simulink model "TST_CoME_DemCoord"  (R2016b)
settings: Solver=FixedStepDiscrete  StartTime=0.0  StopTime=simTime  FixedStep=sampleTime  RelTol=1e-3
values from neighbouring files (symbols this model uses):
  testCase = 1    [initTST_CoME_DemCoord_001.m]    (also in initTST_CoME_DemCoord_002.m = 2; initTST_CoME_DemCoord_003.m = 3; initTST_CoME_DemCoord_004.m = 4)
libraries: simulink x29, UnitTest_Lib x24
(part 1 of 2)
settings Model: Creator=zhengjinyan  LastModifiedBy=zhengjinyan
settings DebuggingCC: SignalRangeChecking=error

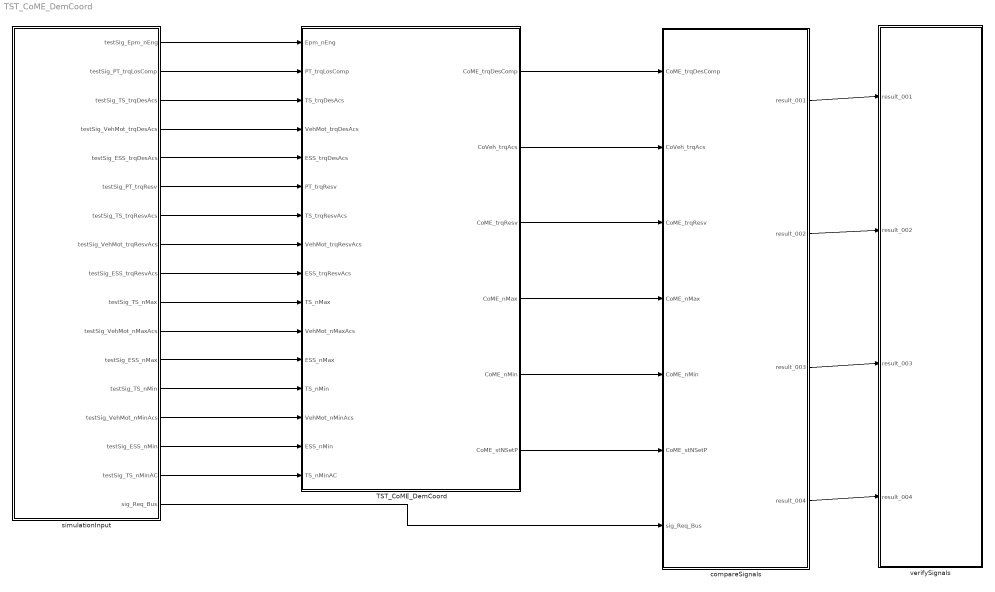
== system TST_CoME_DemCoord ==
  TST_CoME_DemCoord : Subsystem
  compareSignals : Subsystem
  simulationInput : Subsystem
  verifySignals : Subsystem
  wires:
  simulationInput/1(testSig_Epm_nEng) -> TST_CoME_DemCoord/1(Epm_nEng)
  simulationInput/2(testSig_PT_trqLosComp) -> TST_CoME_DemCoord/2(PT_trqLosComp)
  simulationInput/3(testSig_TS_trqDesAcs) -> TST_CoME_DemCoord/3(TS_trqDesAcs)
  simulationInput/4(testSig_VehMot_trqDesAcs) -> TST_CoME_DemCoord/4(VehMot_trqDesAcs)
  simulationInput/5(testSig_ESS_trqDesAcs) -> TST_CoME_DemCoord/5(ESS_trqDesAcs)
  simulationInput/6(testSig_PT_trqResv) -> TST_CoME_DemCoord/6(PT_trqResv)
  simulationInput/7(testSig_TS_trqResvAcs) -> TST_CoME_DemCoord/7(TS_trqResvAcs)
  simulationInput/8(testSig_VehMot_trqResvAcs) -> TST_CoME_DemCoord/8(VehMot_trqResvAcs)
  simulationInput/9(testSig_ESS_trqResvAcs) -> TST_CoME_DemCoord/9(ESS_trqResvAcs)
  simulationInput/10(testSig_TS_nMax) -> TST_CoME_DemCoord/10(TS_nMax)
  simulationInput/11(testSig_VehMot_nMaxAcs) -> TST_CoME_DemCoord/11(VehMot_nMaxAcs)
  simulationInput/12(testSig_ESS_nMax) -> TST_CoME_DemCoord/12(ESS_nMax)
  simulationInput/13(testSig_TS_nMin) -> TST_CoME_DemCoord/13(TS_nMin)
  simulationInput/14(testSig_VehMot_nMinAcs) -> TST_CoME_DemCoord/14(VehMot_nMinAcs)
  simulationInput/15(testSig_ESS_nMin) -> TST_CoME_DemCoord/15(ESS_nMin)
  simulationInput/16(testSig_TS_nMinAC) -> TST_CoME_DemCoord/16(TS_nMinAC)
  TST_CoME_DemCoord/1(CoME_trqDesComp) -> compareSignals/1(CoME_trqDesComp)
  TST_CoME_DemCoord/2(CoVeh_trqAcs) -> compareSignals/2(CoVeh_trqAcs)
  TST_CoME_DemCoord/3(CoME_trqResv) -> compareSignals/3(CoME_trqResv)
  TST_CoME_DemCoord/4(CoME_nMax) -> compareSignals/4(CoME_nMax)
  TST_CoME_DemCoord/5(CoME_nMin) -> compareSignals/5(CoME_nMin)
  TST_CoME_DemCoord/6(CoME_stNSetP) -> compareSignals/6(CoME_stNSetP)
  simulationInput/17(sig_Req_Bus) -> compareSignals/7(sig_Req_Bus)
  compareSignals/1(result_001) -> verifySignals/1(result_001)
  compareSignals/2(result_002) -> verifySignals/2(result_002)
  compareSignals/3(result_003) -> verifySignals/3(result_003)
  compareSignals/4(result_004) -> verifySignals/4(result_004)

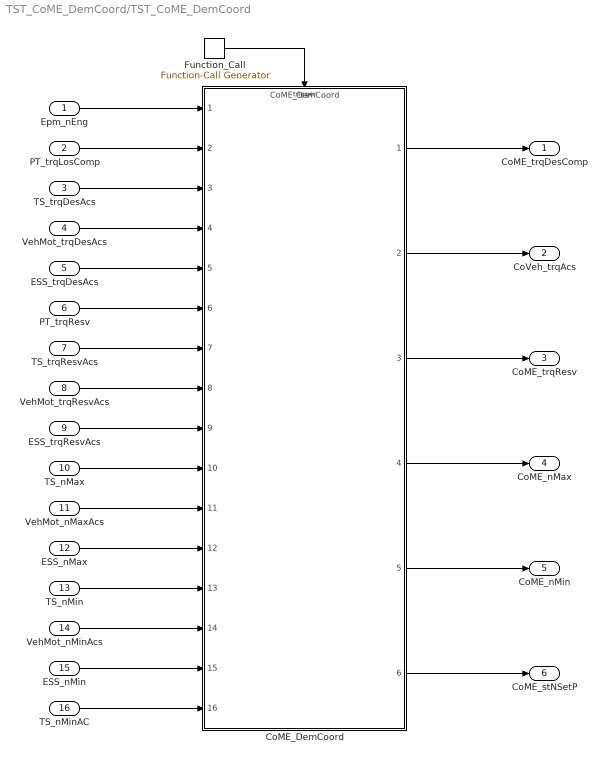
== system TST_CoME_DemCoord/TST_CoME_DemCoord ==
  Epm_nEng : Inport
  PT_trqLosComp : Inport  Port=2
  TS_trqDesAcs : Inport  Port=3
  VehMot_trqDesAcs : Inport  Port=4
  ESS_trqDesAcs : Inport  Port=5
  PT_trqResv : Inport  Port=6
  TS_trqResvAcs : Inport  Port=7
  VehMot_trqResvAcs : Inport  Port=8
  ESS_trqResvAcs : Inport  Port=9
  TS_nMax : Inport  Port=10
  VehMot_nMaxAcs : Inport  Port=11
  ESS_nMax : Inport  Port=12
  TS_nMin : Inport  Port=13
  VehMot_nMinAcs : Inport  Port=14
  ESS_nMin : Inport  Port=15
  TS_nMinAC : Inport  Port=16
  CoME_DemCoord : ModelReference  ModelNameDialog=CoME_DemCoord  SimulationMode=Normal  ModelReferenceVersion=1.11  TriggerPortName=function  TriggerPortTriggerType=function-call  TriggerPortStatesWhenEnabling=held
  Function_Call : simulink/Ports & Subsystems/Function-Call Generator  sample_time=sampleTime  numberOfIterations=1
  CoME_trqDesComp : Outport
  CoVeh_trqAcs : Outport  Port=2
  CoME_trqResv : Outport  Port=3
  CoME_nMax : Outport  Port=4
  CoME_nMin : Outport  Port=5
  CoME_stNSetP : Outport  Port=6
  wires:
  Function_Call/1 -> CoME_DemCoord/Trigger
  Epm_nEng/1 -> CoME_DemCoord/1
  PT_trqLosComp/1 -> CoME_DemCoord/2
  TS_trqDesAcs/1 -> CoME_DemCoord/3
  VehMot_trqDesAcs/1 -> CoME_DemCoord/4
  ESS_trqDesAcs/1 -> CoME_DemCoord/5
  PT_trqResv/1 -> CoME_DemCoord/6
  TS_trqResvAcs/1 -> CoME_DemCoord/7
  VehMot_trqResvAcs/1 -> CoME_DemCoord/8
  ESS_trqResvAcs/1 -> CoME_DemCoord/9
  TS_nMax/1 -> CoME_DemCoord/10
  VehMot_nMaxAcs/1 -> CoME_DemCoord/11
  ESS_nMax/1 -> CoME_DemCoord/12
  TS_nMin/1 -> CoME_DemCoord/13
  VehMot_nMinAcs/1 -> CoME_DemCoord/14
  ESS_nMin/1 -> CoME_DemCoord/15
  TS_nMinAC/1 -> CoME_DemCoord/16
  CoME_DemCoord/1 -> CoME_trqDesComp/1
  CoME_DemCoord/2 -> CoVeh_trqAcs/1
  CoME_DemCoord/3 -> CoME_trqResv/1
  CoME_DemCoord/4 -> CoME_nMax/1
  CoME_DemCoord/5 -> CoME_nMin/1
  CoME_DemCoord/6 -> CoME_stNSetP/1

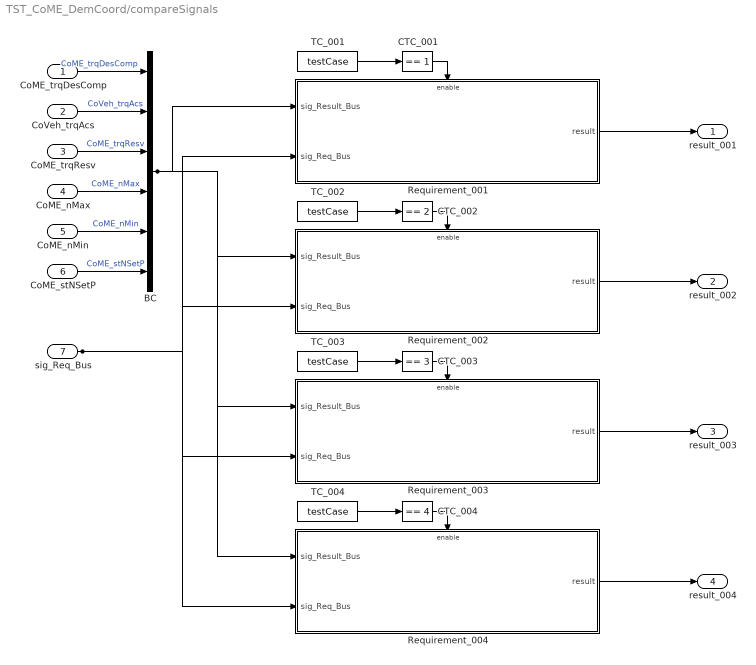
== system TST_CoME_DemCoord/compareSignals ==
  CoME_trqDesComp : Inport
  CoVeh_trqAcs : Inport  Port=2
  CoME_trqResv : Inport  Port=3
  CoME_nMax : Inport  Port=4
  CoME_nMin : Inport  Port=5
  CoME_stNSetP : Inport  Port=6
  sig_Req_Bus : Inport  Port=7
  BC : BusCreator  Inputs=6
  CTC_001 : simulink/Logic and Bit Operations/Compare To Constant  relop===  const=1  OutDataTypeStr=boolean
  CTC_002 : simulink/Logic and Bit Operations/Compare To Constant  relop===  const=2  OutDataTypeStr=boolean
  CTC_003 : simulink/Logic and Bit Operations/Compare To Constant  relop===  const=3  OutDataTypeStr=boolean
  CTC_004 : simulink/Logic and Bit Operations/Compare To Constant  relop===  const=4  OutDataTypeStr=boolean
  Requirement_001 : Subsystem
  Requirement_002 : Subsystem
  Requirement_003 : Subsystem
  Requirement_004 : Subsystem
  TC_001 : Constant  Value=testCase
  TC_002 : Constant  Value=testCase
  TC_003 : Constant  Value=testCase
  TC_004 : Constant  Value=testCase
  result_001 : Outport
  result_002 : Outport  Port=2
  result_003 : Outport  Port=3
  result_004 : Outport  Port=4
  wires:
  CoME_trqDesComp/1 -> BC/1  "CoME_trqDesComp"
  CoVeh_trqAcs/1 -> BC/2  "CoVeh_trqAcs"
  CoME_trqResv/1 -> BC/3  "CoME_trqResv"
  CoME_nMax/1 -> BC/4  "CoME_nMax"
  CoME_nMin/1 -> BC/5  "CoME_nMin"
  CoME_stNSetP/1 -> BC/6  "CoME_stNSetP"
  TC_001/1 -> CTC_001/1
  CTC_001/1 -> Requirement_001/Enable
  sig_Req_Bus/1 -> Requirement_001/2(sig_Req_Bus), Requirement_002/2(sig_Req_Bus), Requirement_003/2(sig_Req_Bus), Requirement_004/2(sig_Req_Bus)
  BC/1 -> Requirement_001/1(sig_Result_Bus), Requirement_002/1(sig_Result_Bus), Requirement_003/1(sig_Result_Bus), Requirement_004/1(sig_Result_Bus)
  Requirement_001/1(result) -> result_001/1
  TC_002/1 -> CTC_002/1
  CTC_002/1 -> Requirement_002/Enable
  Requirement_002/1(result) -> result_002/1
  TC_003/1 -> CTC_003/1
  CTC_003/1 -> Requirement_003/Enable
  Requirement_003/1(result) -> result_003/1
  TC_004/1 -> CTC_004/1
  CTC_004/1 -> Requirement_004/Enable
  Requirement_004/1(result) -> result_004/1

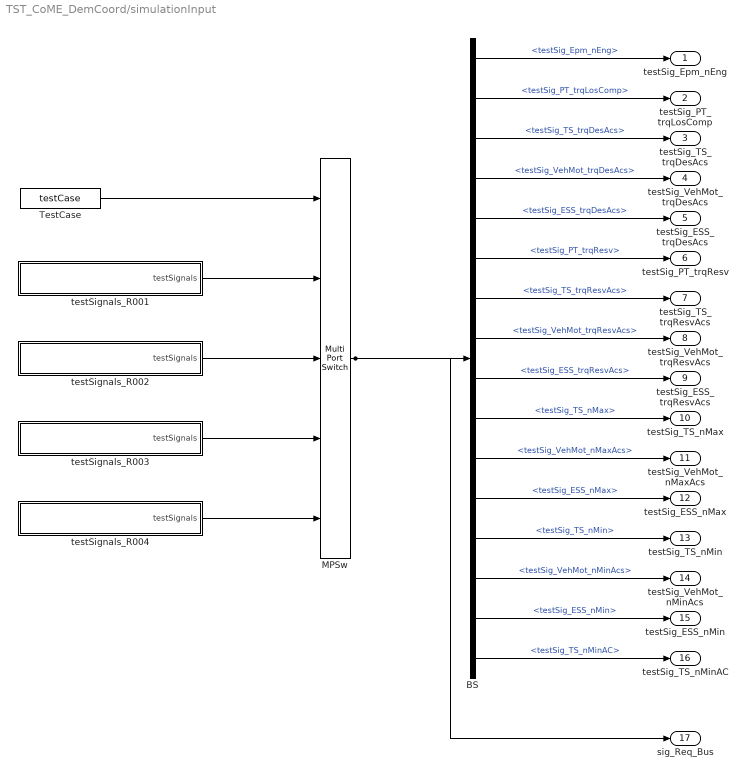
== system TST_CoME_DemCoord/simulationInput ==
  BS : BusSelector  OutputSignals=testSig_Epm_nEng,testSig_PT_trqLosComp,testSig_TS_trqDesAcs,testSig_VehMot_trqDesAcs,testSig_ESS_trqDesAcs,testSig_PT_trqResv,testSig_TS_trqResvAcs,testSig_VehMot_trqResvAcs,testSig_ESS_trqResvAcs,testSig_TS_nMax,testSig_VehMot_nMaxAcs,testSig_ESS_nMax,testSig_TS_nMin,testSig_VehMot_nMinAcs,testSig_ESS_nMin,testSig_TS_nMinAC
  MPSw : MultiPortSwitch  Inputs=4  SaturateOnIntegerOverflow=on  InputSameDT=on
  TestCase : Constant  Value=testCase
  testSignals_R001 : Subsystem
  testSignals_R002 : Subsystem
  testSignals_R003 : Subsystem
  testSignals_R004 : Subsystem
  testSig_Epm_nEng : Outport
  testSig_PT_trqLosComp : Outport  Port=2
  testSig_TS_trqDesAcs : Outport  Port=3
  testSig_VehMot_trqDesAcs : Outport  Port=4
  testSig_ESS_trqDesAcs : Outport  Port=5
  testSig_PT_trqResv : Outport  Port=6
  testSig_TS_trqResvAcs : Outport  Port=7
  testSig_VehMot_trqResvAcs : Outport  Port=8
  testSig_ESS_trqResvAcs : Outport  Port=9
  testSig_TS_nMax : Outport  Port=10
  testSig_VehMot_nMaxAcs : Outport  Port=11
  testSig_ESS_nMax : Outport  Port=12
  testSig_TS_nMin : Outport  Port=13
  testSig_VehMot_nMinAcs : Outport  Port=14
  testSig_ESS_nMin : Outport  Port=15
  testSig_TS_nMinAC : Outport  Port=16
  sig_Req_Bus : Outport  Port=17
  wires:
  BS/1 -> testSig_Epm_nEng/1  "<testSig_Epm_nEng>"
  BS/2 -> testSig_PT_trqLosComp/1  "<testSig_PT_trqLosComp>"
  BS/3 -> testSig_TS_trqDesAcs/1  "<testSig_TS_trqDesAcs>"
  BS/4 -> testSig_VehMot_trqDesAcs/1  "<testSig_VehMot_trqDesAcs>"
  BS/5 -> testSig_ESS_trqDesAcs/1  "<testSig_ESS_trqDesAcs>"
  BS/6 -> testSig_PT_trqResv/1  "<testSig_PT_trqResv>"
  BS/7 -> testSig_TS_trqResvAcs/1  "<testSig_TS_trqResvAcs>"
  BS/8 -> testSig_VehMot_trqResvAcs/1  "<testSig_VehMot_trqResvAcs>"
  BS/9 -> testSig_ESS_trqResvAcs/1  "<testSig_ESS_trqResvAcs>"
  BS/10 -> testSig_TS_nMax/1  "<testSig_TS_nMax>"
  BS/11 -> testSig_VehMot_nMaxAcs/1  "<testSig_VehMot_nMaxAcs>"
  BS/12 -> testSig_ESS_nMax/1  "<testSig_ESS_nMax>"
  BS/13 -> testSig_TS_nMin/1  "<testSig_TS_nMin>"
  BS/14 -> testSig_VehMot_nMinAcs/1  "<testSig_VehMot_nMinAcs>"
  BS/15 -> testSig_ESS_nMin/1  "<testSig_ESS_nMin>"
  BS/16 -> testSig_TS_nMinAC/1  "<testSig_TS_nMinAC>"
  MPSw/1 -> BS/1, sig_Req_Bus/1
  TestCase/1 -> MPSw/1
  testSignals_R001/1(testSignals) -> MPSw/2
  testSignals_R002/1(testSignals) -> MPSw/3
  testSignals_R003/1(testSignals) -> MPSw/4
  testSignals_R004/1(testSignals) -> MPSw/5

== system TST_CoME_DemCoord/verifySignals ==
  result_001 : Inport
  result_002 : Inport  Port=2
  result_003 : Inport  Port=3
  result_004 : Inport  Port=4
  Assertion_001 : Assertion  Enabled=off
  Assertion_002 : Assertion  Enabled=off
  Assertion_003 : Assertion  Enabled=off
  Assertion_004 : Assertion  Enabled=off
  wires:
  result_001/1 -> Assertion_001/1
  result_002/1 -> Assertion_002/1
  result_003/1 -> Assertion_003/1
  result_004/1 -> Assertion_004/1

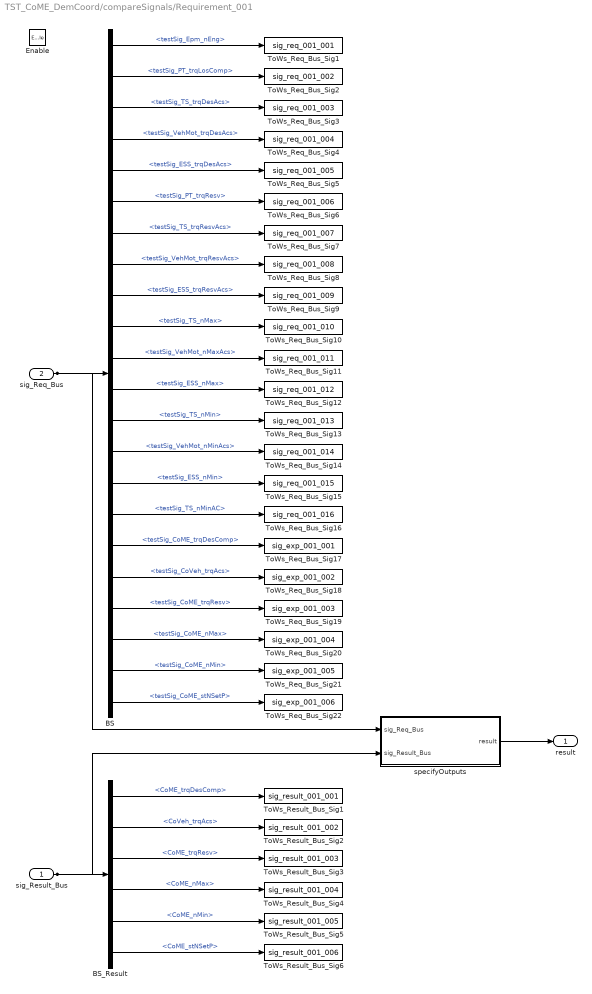
== system TST_CoME_DemCoord/compareSignals/Requirement_001 ==
  sig_Result_Bus : Inport
  sig_Req_Bus : Inport  Port=2
  Enable : EnablePort
  BS : BusSelector  OutputSignals=testSig_Epm_nEng,testSig_PT_trqLosComp,testSig_TS_trqDesAcs,testSig_VehMot_trqDesAcs,testSig_ESS_trqDesAcs,testSig_PT_trqResv,testSig_TS_trqResvAcs,testSig_VehMot_trqResvAcs,testSig_ESS_trqResvAcs,testSig_TS_nMax,testSig_VehMot_nMaxAcs,testSig_ESS_nMax,testSig_TS_nMin,testSig_VehMot_nMinAcs,testSig_ESS_nMin,testSig_TS_nMinAC,testSig_CoME_trqDesComp,testSig_CoVeh_trqAcs,testSig_CoME_trqResv,testSig_CoME_nMax,testSig_CoME_nMin,testSig_CoME_stNSetP
  BS_Result : BusSelector  OutputSignals=CoME_trqDesComp,CoVeh_trqAcs,CoME_trqResv,CoME_nMax,CoME_nMin,CoME_stNSetP
  ToWs_Req_Bus_Sig1 : ToWorkspace  VariableName=sig_req_001_001  SaveFormat=Structure With Time
  ToWs_Req_Bus_Sig10 : ToWorkspace  VariableName=sig_req_001_010  SaveFormat=Structure With Time
  ToWs_Req_Bus_Sig11 : ToWorkspace  VariableName=sig_req_001_011  SaveFormat=Structure With Time
  ToWs_Req_Bus_Sig12 : ToWorkspace  VariableName=sig_req_001_012  SaveFormat=Structure With Time
  ToWs_Req_Bus_Sig13 : ToWorkspace  VariableName=sig_req_001_013  SaveFormat=Structure With Time
  ToWs_Req_Bus_Sig14 : ToWorkspace  VariableName=sig_req_001_014  SaveFormat=Structure With Time
  ToWs_Req_Bus_Sig15 : ToWorkspace  VariableName=sig_req_001_015  SaveFormat=Structure With Time
  ToWs_Req_Bus_Sig16 : ToWorkspace  VariableName=sig_req_001_016  SaveFormat=Structure With Time
  ToWs_Req_Bus_Sig17 : ToWorkspace  VariableName=sig_exp_001_001  SaveFormat=Structure With Time
  ToWs_Req_Bus_Sig18 : ToWorkspace  VariableName=sig_exp_001_002  SaveFormat=Structure With Time
  ToWs_Req_Bus_Sig19 : ToWorkspace  VariableName=sig_exp_001_003  SaveFormat=Structure With Time
  ToWs_Req_Bus_Sig2 : ToWorkspace  VariableName=sig_req_001_002  SaveFormat=Structure With Time
  ToWs_Req_Bus_Sig20 : ToWorkspace  VariableName=sig_exp_001_004  SaveFormat=Structure With Time
  ToWs_Req_Bus_Sig21 : ToWorkspace  VariableName=sig_exp_001_005  SaveFormat=Structure With Time
  ToWs_Req_Bus_Sig22 : ToWorkspace  VariableName=sig_exp_001_006  SaveFormat=Structure With Time
  ToWs_Req_Bus_Sig3 : ToWorkspace  VariableName=sig_req_001_003  SaveFormat=Structure With Time
  ToWs_Req_Bus_Sig4 : ToWorkspace  VariableName=sig_req_001_004  SaveFormat=Structure With Time
  ToWs_Req_Bus_Sig5 : ToWorkspace  VariableName=sig_req_001_005  SaveFormat=Structure With Time
  ToWs_Req_Bus_Sig6 : ToWorkspace  VariableName=sig_req_001_006  SaveFormat=Structure With Time
  ToWs_Req_Bus_Sig7 : ToWorkspace  VariableName=sig_req_001_007  SaveFormat=Structure With Time
  ToWs_Req_Bus_Sig8 : ToWorkspace  VariableName=sig_req_001_008  SaveFormat=Structure With Time
  ToWs_Req_Bus_Sig9 : ToWorkspace  VariableName=sig_req_001_009  SaveFormat=Structure With Time
  ToWs_Result_Bus_Sig1 : ToWorkspace  VariableName=sig_result_001_001  SaveFormat=Structure With Time
  ToWs_Result_Bus_Sig2 : ToWorkspace  VariableName=sig_result_001_002  SaveFormat=Structure With Time
  ToWs_Result_Bus_Sig3 : ToWorkspace  VariableName=sig_result_001_003  SaveFormat=Structure With Time
  ToWs_Result_Bus_Sig4 : ToWorkspace  VariableName=sig_result_001_004  SaveFormat=Structure With Time
  ToWs_Result_Bus_Sig5 : ToWorkspace  VariableName=sig_result_001_005  SaveFormat=Structure With Time
  ToWs_Result_Bus_Sig6 : ToWorkspace  VariableName=sig_result_001_006  SaveFormat=Structure With Time
  specifyOutputs : Subsystem
  result : Outport
  wires:
  sig_Req_Bus/1 -> BS/1, specifyOutputs/1(sig_Req_Bus)
  BS/1 -> ToWs_Req_Bus_Sig1/1  "<testSig_Epm_nEng>"
  BS/2 -> ToWs_Req_Bus_Sig2/1  "<testSig_PT_trqLosComp>"
  BS/3 -> ToWs_Req_Bus_Sig3/1  "<testSig_TS_trqDesAcs>"
  BS/4 -> ToWs_Req_Bus_Sig4/1  "<testSig_VehMot_trqDesAcs>"
  BS/5 -> ToWs_Req_Bus_Sig5/1  "<testSig_ESS_trqDesAcs>"
  BS/6 -> ToWs_Req_Bus_Sig6/1  "<testSig_PT_trqResv>"
  BS/7 -> ToWs_Req_Bus_Sig7/1  "<testSig_TS_trqResvAcs>"
  BS/8 -> ToWs_Req_Bus_Sig8/1  "<testSig_VehMot_trqResvAcs>"
  BS/9 -> ToWs_Req_Bus_Sig9/1  "<testSig_ESS_trqResvAcs>"
  BS/10 -> ToWs_Req_Bus_Sig10/1  "<testSig_TS_nMax>"
  BS/11 -> ToWs_Req_Bus_Sig11/1  "<testSig_VehMot_nMaxAcs>"
  BS/12 -> ToWs_Req_Bus_Sig12/1  "<testSig_ESS_nMax>"
  BS/13 -> ToWs_Req_Bus_Sig13/1  "<testSig_TS_nMin>"
  BS/14 -> ToWs_Req_Bus_Sig14/1  "<testSig_VehMot_nMinAcs>"
  BS/15 -> ToWs_Req_Bus_Sig15/1  "<testSig_ESS_nMin>"
  BS/16 -> ToWs_Req_Bus_Sig16/1  "<testSig_TS_nMinAC>"
  BS/17 -> ToWs_Req_Bus_Sig17/1  "<testSig_CoME_trqDesComp>"
  BS/18 -> ToWs_Req_Bus_Sig18/1  "<testSig_CoVeh_trqAcs>"
  BS/19 -> ToWs_Req_Bus_Sig19/1  "<testSig_CoME_trqResv>"
  BS/20 -> ToWs_Req_Bus_Sig20/1  "<testSig_CoME_nMax>"
  BS/21 -> ToWs_Req_Bus_Sig21/1  "<testSig_CoME_nMin>"
  BS/22 -> ToWs_Req_Bus_Sig22/1  "<testSig_CoME_stNSetP>"
  sig_Result_Bus/1 -> BS_Result/1, specifyOutputs/2(sig_Result_Bus)
  BS_Result/1 -> ToWs_Result_Bus_Sig1/1  "<CoME_trqDesComp>"
  BS_Result/2 -> ToWs_Result_Bus_Sig2/1  "<CoVeh_trqAcs>"
  BS_Result/3 -> ToWs_Result_Bus_Sig3/1  "<CoME_trqResv>"
  BS_Result/4 -> ToWs_Result_Bus_Sig4/1  "<CoME_nMax>"
  BS_Result/5 -> ToWs_Result_Bus_Sig5/1  "<CoME_nMin>"
  BS_Result/6 -> ToWs_Result_Bus_Sig6/1  "<CoME_stNSetP>"
  specifyOutputs/1(result) -> result/1

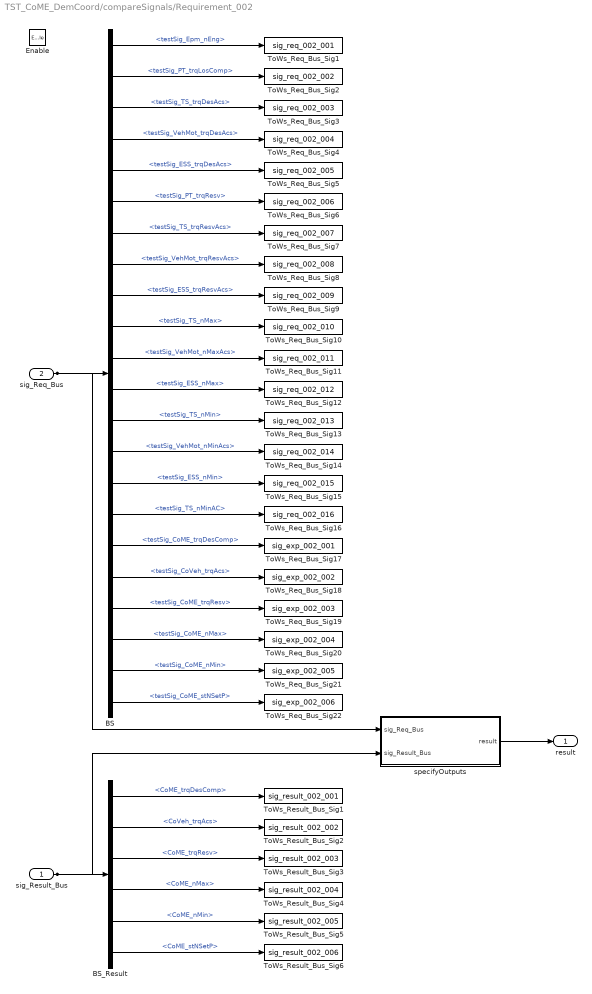
== system TST_CoME_DemCoord/compareSignals/Requirement_002 ==
  sig_Result_Bus : Inport
  sig_Req_Bus : Inport  Port=2
  Enable : EnablePort
  BS : BusSelector  OutputSignals=testSig_Epm_nEng,testSig_PT_trqLosComp,testSig_TS_trqDesAcs,testSig_VehMot_trqDesAcs,testSig_ESS_trqDesAcs,testSig_PT_trqResv,testSig_TS_trqResvAcs,testSig_VehMot_trqResvAcs,testSig_ESS_trqResvAcs,testSig_TS_nMax,testSig_VehMot_nMaxAcs,testSig_ESS_nMax,testSig_TS_nMin,testSig_VehMot_nMinAcs,testSig_ESS_nMin,testSig_TS_nMinAC,testSig_CoME_trqDesComp,testSig_CoVeh_trqAcs,testSig_CoME_trqResv,testSig_CoME_nMax,testSig_CoME_nMin,testSig_CoME_stNSetP
  BS_Result : BusSelector  OutputSignals=CoME_trqDesComp,CoVeh_trqAcs,CoME_trqResv,CoME_nMax,CoME_nMin,CoME_stNSetP
  ToWs_Req_Bus_Sig1 : ToWorkspace  VariableName=sig_req_002_001  SaveFormat=Structure With Time
  ToWs_Req_Bus_Sig10 : ToWorkspace  VariableName=sig_req_002_010  SaveFormat=Structure With Time
  ToWs_Req_Bus_Sig11 : ToWorkspace  VariableName=sig_req_002_011  SaveFormat=Structure With Time
  ToWs_Req_Bus_Sig12 : ToWorkspace  VariableName=sig_req_002_012  SaveFormat=Structure With Time
  ToWs_Req_Bus_Sig13 : ToWorkspace  VariableName=sig_req_002_013  SaveFormat=Structure With Time
  ToWs_Req_Bus_Sig14 : ToWorkspace  VariableName=sig_req_002_014  SaveFormat=Structure With Time
  ToWs_Req_Bus_Sig15 : ToWorkspace  VariableName=sig_req_002_015  SaveFormat=Structure With Time
  ToWs_Req_Bus_Sig16 : ToWorkspace  VariableName=sig_req_002_016  SaveFormat=Structure With Time
  ToWs_Req_Bus_Sig17 : ToWorkspace  VariableName=sig_exp_002_001  SaveFormat=Structure With Time
  ToWs_Req_Bus_Sig18 : ToWorkspace  VariableName=sig_exp_002_002  SaveFormat=Structure With Time
  ToWs_Req_Bus_Sig19 : ToWorkspace  VariableName=sig_exp_002_003  SaveFormat=Structure With Time
  ToWs_Req_Bus_Sig2 : ToWorkspace  VariableName=sig_req_002_002  SaveFormat=Structure With Time
  ToWs_Req_Bus_Sig20 : ToWorkspace  VariableName=sig_exp_002_004  SaveFormat=Structure With Time
  ToWs_Req_Bus_Sig21 : ToWorkspace  VariableName=sig_exp_002_005  SaveFormat=Structure With Time
  ToWs_Req_Bus_Sig22 : ToWorkspace  VariableName=sig_exp_002_006  SaveFormat=Structure With Time
  ToWs_Req_Bus_Sig3 : ToWorkspace  VariableName=sig_req_002_003  SaveFormat=Structure With Time
  ToWs_Req_Bus_Sig4 : ToWorkspace  VariableName=sig_req_002_004  SaveFormat=Structure With Time
  ToWs_Req_Bus_Sig5 : ToWorkspace  VariableName=sig_req_002_005  SaveFormat=Structure With Time
  ToWs_Req_Bus_Sig6 : ToWorkspace  VariableName=sig_req_002_006  SaveFormat=Structure With Time
  ToWs_Req_Bus_Sig7 : ToWorkspace  VariableName=sig_req_002_007  SaveFormat=Structure With Time
  ToWs_Req_Bus_Sig8 : ToWorkspace  VariableName=sig_req_002_008  SaveFormat=Structure With Time
  ToWs_Req_Bus_Sig9 : ToWorkspace  VariableName=sig_req_002_009  SaveFormat=Structure With Time
  ToWs_Result_Bus_Sig1 : ToWorkspace  VariableName=sig_result_002_001  SaveFormat=Structure With Time
  ToWs_Result_Bus_Sig2 : ToWorkspace  VariableName=sig_result_002_002  SaveFormat=Structure With Time
  ToWs_Result_Bus_Sig3 : ToWorkspace  VariableName=sig_result_002_003  SaveFormat=Structure With Time
  ToWs_Result_Bus_Sig4 : ToWorkspace  VariableName=sig_result_002_004  SaveFormat=Structure With Time
  ToWs_Result_Bus_Sig5 : ToWorkspace  VariableName=sig_result_002_005  SaveFormat=Structure With Time
  ToWs_Result_Bus_Sig6 : ToWorkspace  VariableName=sig_result_002_006  SaveFormat=Structure With Time
  specifyOutputs : Subsystem
  result : Outport
  wires:
  sig_Req_Bus/1 -> BS/1, specifyOutputs/1(sig_Req_Bus)
  BS/1 -> ToWs_Req_Bus_Sig1/1  "<testSig_Epm_nEng>"
  BS/2 -> ToWs_Req_Bus_Sig2/1  "<testSig_PT_trqLosComp>"
  BS/3 -> ToWs_Req_Bus_Sig3/1  "<testSig_TS_trqDesAcs>"
  BS/4 -> ToWs_Req_Bus_Sig4/1  "<testSig_VehMot_trqDesAcs>"
  BS/5 -> ToWs_Req_Bus_Sig5/1  "<testSig_ESS_trqDesAcs>"
  BS/6 -> ToWs_Req_Bus_Sig6/1  "<testSig_PT_trqResv>"
  BS/7 -> ToWs_Req_Bus_Sig7/1  "<testSig_TS_trqResvAcs>"
  BS/8 -> ToWs_Req_Bus_Sig8/1  "<testSig_VehMot_trqResvAcs>"
  BS/9 -> ToWs_Req_Bus_Sig9/1  "<testSig_ESS_trqResvAcs>"
  BS/10 -> ToWs_Req_Bus_Sig10/1  "<testSig_TS_nMax>"
  BS/11 -> ToWs_Req_Bus_Sig11/1  "<testSig_VehMot_nMaxAcs>"
  BS/12 -> ToWs_Req_Bus_Sig12/1  "<testSig_ESS_nMax>"
  BS/13 -> ToWs_Req_Bus_Sig13/1  "<testSig_TS_nMin>"
  BS/14 -> ToWs_Req_Bus_Sig14/1  "<testSig_VehMot_nMinAcs>"
  BS/15 -> ToWs_Req_Bus_Sig15/1  "<testSig_ESS_nMin>"
  BS/16 -> ToWs_Req_Bus_Sig16/1  "<testSig_TS_nMinAC>"
  BS/17 -> ToWs_Req_Bus_Sig17/1  "<testSig_CoME_trqDesComp>"
  BS/18 -> ToWs_Req_Bus_Sig18/1  "<testSig_CoVeh_trqAcs>"
  BS/19 -> ToWs_Req_Bus_Sig19/1  "<testSig_CoME_trqResv>"
  BS/20 -> ToWs_Req_Bus_Sig20/1  "<testSig_CoME_nMax>"
  BS/21 -> ToWs_Req_Bus_Sig21/1  "<testSig_CoME_nMin>"
  BS/22 -> ToWs_Req_Bus_Sig22/1  "<testSig_CoME_stNSetP>"
  sig_Result_Bus/1 -> BS_Result/1, specifyOutputs/2(sig_Result_Bus)
  BS_Result/1 -> ToWs_Result_Bus_Sig1/1  "<CoME_trqDesComp>"
  BS_Result/2 -> ToWs_Result_Bus_Sig2/1  "<CoVeh_trqAcs>"
  BS_Result/3 -> ToWs_Result_Bus_Sig3/1  "<CoME_trqResv>"
  BS_Result/4 -> ToWs_Result_Bus_Sig4/1  "<CoME_nMax>"
  BS_Result/5 -> ToWs_Result_Bus_Sig5/1  "<CoME_nMin>"
  BS_Result/6 -> ToWs_Result_Bus_Sig6/1  "<CoME_stNSetP>"
  specifyOutputs/1(result) -> result/1

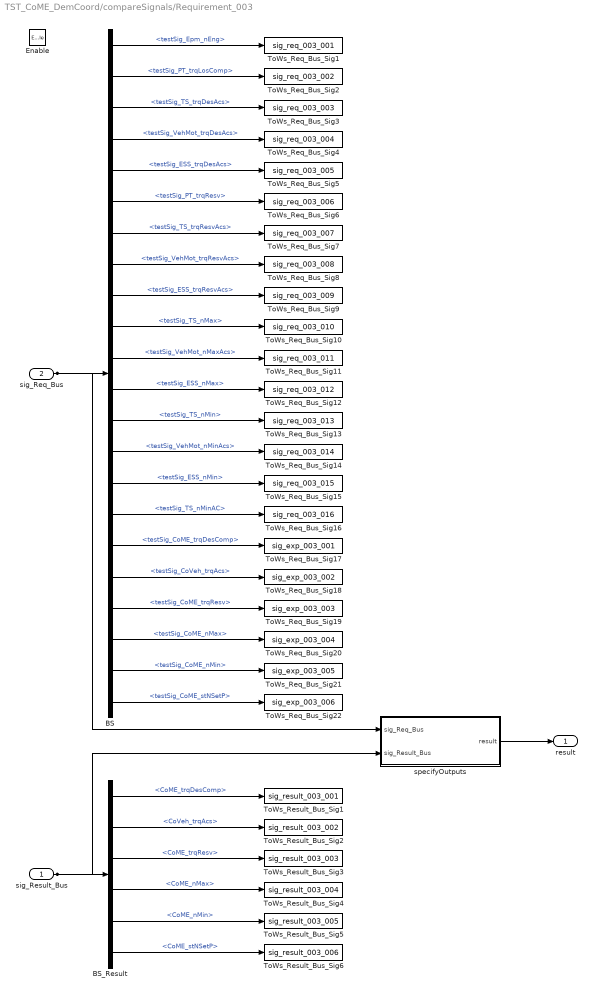
== system TST_CoME_DemCoord/compareSignals/Requirement_003 ==
  sig_Result_Bus : Inport
  sig_Req_Bus : Inport  Port=2
  Enable : EnablePort
  BS : BusSelector  OutputSignals=testSig_Epm_nEng,testSig_PT_trqLosComp,testSig_TS_trqDesAcs,testSig_VehMot_trqDesAcs,testSig_ESS_trqDesAcs,testSig_PT_trqResv,testSig_TS_trqResvAcs,testSig_VehMot_trqResvAcs,testSig_ESS_trqResvAcs,testSig_TS_nMax,testSig_VehMot_nMaxAcs,testSig_ESS_nMax,testSig_TS_nMin,testSig_VehMot_nMinAcs,testSig_ESS_nMin,testSig_TS_nMinAC,testSig_CoME_trqDesComp,testSig_CoVeh_trqAcs,testSig_CoME_trqResv,testSig_CoME_nMax,testSig_CoME_nMin,testSig_CoME_stNSetP
  BS_Result : BusSelector  OutputSignals=CoME_trqDesComp,CoVeh_trqAcs,CoME_trqResv,CoME_nMax,CoME_nMin,CoME_stNSetP
  ToWs_Req_Bus_Sig1 : ToWorkspace  VariableName=sig_req_003_001  SaveFormat=Structure With Time
  ToWs_Req_Bus_Sig10 : ToWorkspace  VariableName=sig_req_003_010  SaveFormat=Structure With Time
  ToWs_Req_Bus_Sig11 : ToWorkspace  VariableName=sig_req_003_011  SaveFormat=Structure With Time
  ToWs_Req_Bus_Sig12 : ToWorkspace  VariableName=sig_req_003_012  SaveFormat=Structure With Time
  ToWs_Req_Bus_Sig13 : ToWorkspace  VariableName=sig_req_003_013  SaveFormat=Structure With Time
  ToWs_Req_Bus_Sig14 : ToWorkspace  VariableName=sig_req_003_014  SaveFormat=Structure With Time
  ToWs_Req_Bus_Sig15 : ToWorkspace  VariableName=sig_req_003_015  SaveFormat=Structure With Time
  ToWs_Req_Bus_Sig16 : ToWorkspace  VariableName=sig_req_003_016  SaveFormat=Structure With Time
  ToWs_Req_Bus_Sig17 : ToWorkspace  VariableName=sig_exp_003_001  SaveFormat=Structure With Time
  ToWs_Req_Bus_Sig18 : ToWorkspace  VariableName=sig_exp_003_002  SaveFormat=Structure With Time
  ToWs_Req_Bus_Sig19 : ToWorkspace  VariableName=sig_exp_003_003  SaveFormat=Structure With Time
  ToWs_Req_Bus_Sig2 : ToWorkspace  VariableName=sig_req_003_002  SaveFormat=Structure With Time
  ToWs_Req_Bus_Sig20 : ToWorkspace  VariableName=sig_exp_003_004  SaveFormat=Structure With Time
  ToWs_Req_Bus_Sig21 : ToWorkspace  VariableName=sig_exp_003_005  SaveFormat=Structure With Time
  ToWs_Req_Bus_Sig22 : ToWorkspace  VariableName=sig_exp_003_006  SaveFormat=Structure With Time
  ToWs_Req_Bus_Sig3 : ToWorkspace  VariableName=sig_req_003_003  SaveFormat=Structure With Time
  ToWs_Req_Bus_Sig4 : ToWorkspace  VariableName=sig_req_003_004  SaveFormat=Structure With Time
  ToWs_Req_Bus_Sig5 : ToWorkspace  VariableName=sig_req_003_005  SaveFormat=Structure With Time
  ToWs_Req_Bus_Sig6 : ToWorkspace  VariableName=sig_req_003_006  SaveFormat=Structure With Time
  ToWs_Req_Bus_Sig7 : ToWorkspace  VariableName=sig_req_003_007  SaveFormat=Structure With Time
  ToWs_Req_Bus_Sig8 : ToWorkspace  VariableName=sig_req_003_008  SaveFormat=Structure With Time
  ToWs_Req_Bus_Sig9 : ToWorkspace  VariableName=sig_req_003_009  SaveFormat=Structure With Time
  ToWs_Result_Bus_Sig1 : ToWorkspace  VariableName=sig_result_003_001  SaveFormat=Structure With Time
  ToWs_Result_Bus_Sig2 : ToWorkspace  VariableName=sig_result_003_002  SaveFormat=Structure With Time
  ToWs_Result_Bus_Sig3 : ToWorkspace  VariableName=sig_result_003_003  SaveFormat=Structure With Time
  ToWs_Result_Bus_Sig4 : ToWorkspace  VariableName=sig_result_003_004  SaveFormat=Structure With Time
  ToWs_Result_Bus_Sig5 : ToWorkspace  VariableName=sig_result_003_005  SaveFormat=Structure With Time
  ToWs_Result_Bus_Sig6 : ToWorkspace  VariableName=sig_result_003_006  SaveFormat=Structure With Time
  specifyOutputs : Subsystem
  result : Outport
  wires:
  sig_Req_Bus/1 -> BS/1, specifyOutputs/1(sig_Req_Bus)
  BS/1 -> ToWs_Req_Bus_Sig1/1  "<testSig_Epm_nEng>"
  BS/2 -> ToWs_Req_Bus_Sig2/1  "<testSig_PT_trqLosComp>"
  BS/3 -> ToWs_Req_Bus_Sig3/1  "<testSig_TS_trqDesAcs>"
  BS/4 -> ToWs_Req_Bus_Sig4/1  "<testSig_VehMot_trqDesAcs>"
  BS/5 -> ToWs_Req_Bus_Sig5/1  "<testSig_ESS_trqDesAcs>"
  BS/6 -> ToWs_Req_Bus_Sig6/1  "<testSig_PT_trqResv>"
  BS/7 -> ToWs_Req_Bus_Sig7/1  "<testSig_TS_trqResvAcs>"
  BS/8 -> ToWs_Req_Bus_Sig8/1  "<testSig_VehMot_trqResvAcs>"
  BS/9 -> ToWs_Req_Bus_Sig9/1  "<testSig_ESS_trqResvAcs>"
  BS/10 -> ToWs_Req_Bus_Sig10/1  "<testSig_TS_nMax>"
  BS/11 -> ToWs_Req_Bus_Sig11/1  "<testSig_VehMot_nMaxAcs>"
  BS/12 -> ToWs_Req_Bus_Sig12/1  "<testSig_ESS_nMax>"
  BS/13 -> ToWs_Req_Bus_Sig13/1  "<testSig_TS_nMin>"
  BS/14 -> ToWs_Req_Bus_Sig14/1  "<testSig_VehMot_nMinAcs>"
  BS/15 -> ToWs_Req_Bus_Sig15/1  "<testSig_ESS_nMin>"
  BS/16 -> ToWs_Req_Bus_Sig16/1  "<testSig_TS_nMinAC>"
  BS/17 -> ToWs_Req_Bus_Sig17/1  "<testSig_CoME_trqDesComp>"
  BS/18 -> ToWs_Req_Bus_Sig18/1  "<testSig_CoVeh_trqAcs>"
  BS/19 -> ToWs_Req_Bus_Sig19/1  "<testSig_CoME_trqResv>"
  BS/20 -> ToWs_Req_Bus_Sig20/1  "<testSig_CoME_nMax>"
  BS/21 -> ToWs_Req_Bus_Sig21/1  "<testSig_CoME_nMin>"
  BS/22 -> ToWs_Req_Bus_Sig22/1  "<testSig_CoME_stNSetP>"
  sig_Result_Bus/1 -> BS_Result/1, specifyOutputs/2(sig_Result_Bus)
  BS_Result/1 -> ToWs_Result_Bus_Sig1/1  "<CoME_trqDesComp>"
  BS_Result/2 -> ToWs_Result_Bus_Sig2/1  "<CoVeh_trqAcs>"
  BS_Result/3 -> ToWs_Result_Bus_Sig3/1  "<CoME_trqResv>"
  BS_Result/4 -> ToWs_Result_Bus_Sig4/1  "<CoME_nMax>"
  BS_Result/5 -> ToWs_Result_Bus_Sig5/1  "<CoME_nMin>"
  BS_Result/6 -> ToWs_Result_Bus_Sig6/1  "<CoME_stNSetP>"
  specifyOutputs/1(result) -> result/1

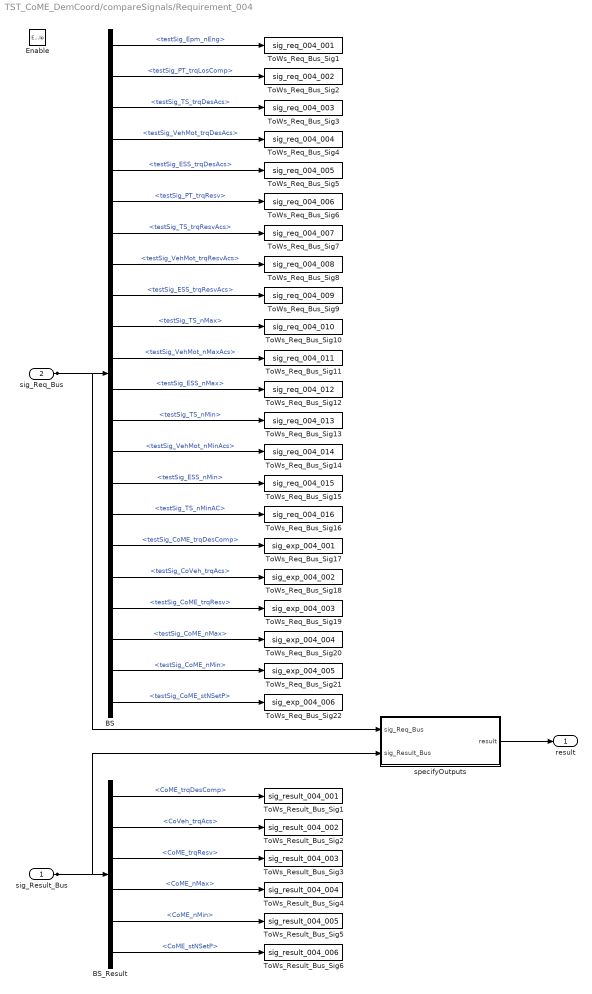
== system TST_CoME_DemCoord/compareSignals/Requirement_004 ==
  sig_Result_Bus : Inport
  sig_Req_Bus : Inport  Port=2
  Enable : EnablePort
  BS : BusSelector  OutputSignals=testSig_Epm_nEng,testSig_PT_trqLosComp,testSig_TS_trqDesAcs,testSig_VehMot_trqDesAcs,testSig_ESS_trqDesAcs,testSig_PT_trqResv,testSig_TS_trqResvAcs,testSig_VehMot_trqResvAcs,testSig_ESS_trqResvAcs,testSig_TS_nMax,testSig_VehMot_nMaxAcs,testSig_ESS_nMax,testSig_TS_nMin,testSig_VehMot_nMinAcs,testSig_ESS_nMin,testSig_TS_nMinAC,testSig_CoME_trqDesComp,testSig_CoVeh_trqAcs,testSig_CoME_trqResv,testSig_CoME_nMax,testSig_CoME_nMin,testSig_CoME_stNSetP
  BS_Result : BusSelector  OutputSignals=CoME_trqDesComp,CoVeh_trqAcs,CoME_trqResv,CoME_nMax,CoME_nMin,CoME_stNSetP
  ToWs_Req_Bus_Sig1 : ToWorkspace  VariableName=sig_req_004_001  SaveFormat=Structure With Time
  ToWs_Req_Bus_Sig10 : ToWorkspace  VariableName=sig_req_004_010  SaveFormat=Structure With Time
  ToWs_Req_Bus_Sig11 : ToWorkspace  VariableName=sig_req_004_011  SaveFormat=Structure With Time
  ToWs_Req_Bus_Sig12 : ToWorkspace  VariableName=sig_req_004_012  SaveFormat=Structure With Time
  ToWs_Req_Bus_Sig13 : ToWorkspace  VariableName=sig_req_004_013  SaveFormat=Structure With Time
  ToWs_Req_Bus_Sig14 : ToWorkspace  VariableName=sig_req_004_014  SaveFormat=Structure With Time
  ToWs_Req_Bus_Sig15 : ToWorkspace  VariableName=sig_req_004_015  SaveFormat=Structure With Time
  ToWs_Req_Bus_Sig16 : ToWorkspace  VariableName=sig_req_004_016  SaveFormat=Structure With Time
  ToWs_Req_Bus_Sig17 : ToWorkspace  VariableName=sig_exp_004_001  SaveFormat=Structure With Time
  ToWs_Req_Bus_Sig18 : ToWorkspace  VariableName=sig_exp_004_002  SaveFormat=Structure With Time
  ToWs_Req_Bus_Sig19 : ToWorkspace  VariableName=sig_exp_004_003  SaveFormat=Structure With Time
  ToWs_Req_Bus_Sig2 : ToWorkspace  VariableName=sig_req_004_002  SaveFormat=Structure With Time
  ToWs_Req_Bus_Sig20 : ToWorkspace  VariableName=sig_exp_004_004  SaveFormat=Structure With Time
  ToWs_Req_Bus_Sig21 : ToWorkspace  VariableName=sig_exp_004_005  SaveFormat=Structure With Time
  ToWs_Req_Bus_Sig22 : ToWorkspace  VariableName=sig_exp_004_006  SaveFormat=Structure With Time
  ToWs_Req_Bus_Sig3 : ToWorkspace  VariableName=sig_req_004_003  SaveFormat=Structure With Time
  ToWs_Req_Bus_Sig4 : ToWorkspace  VariableName=sig_req_004_004  SaveFormat=Structure With Time
  ToWs_Req_Bus_Sig5 : ToWorkspace  VariableName=sig_req_004_005  SaveFormat=Structure With Time
  ToWs_Req_Bus_Sig6 : ToWorkspace  VariableName=sig_req_004_006  SaveFormat=Structure With Time
  ToWs_Req_Bus_Sig7 : ToWorkspace  VariableName=sig_req_004_007  SaveFormat=Structure With Time
  ToWs_Req_Bus_Sig8 : ToWorkspace  VariableName=sig_req_004_008  SaveFormat=Structure With Time
  ToWs_Req_Bus_Sig9 : ToWorkspace  VariableName=sig_req_004_009  SaveFormat=Structure With Time
  ToWs_Result_Bus_Sig1 : ToWorkspace  VariableName=sig_result_004_001  SaveFormat=Structure With Time
  ToWs_Result_Bus_Sig2 : ToWorkspace  VariableName=sig_result_004_002  SaveFormat=Structure With Time
  ToWs_Result_Bus_Sig3 : ToWorkspace  VariableName=sig_result_004_003  SaveFormat=Structure With Time
  ToWs_Result_Bus_Sig4 : ToWorkspace  VariableName=sig_result_004_004  SaveFormat=Structure With Time
  ToWs_Result_Bus_Sig5 : ToWorkspace  VariableName=sig_result_004_005  SaveFormat=Structure With Time
  ToWs_Result_Bus_Sig6 : ToWorkspace  VariableName=sig_result_004_006  SaveFormat=Structure With Time
  specifyOutputs : Subsystem
  result : Outport
  wires:
  sig_Req_Bus/1 -> BS/1, specifyOutputs/1(sig_Req_Bus)
  BS/1 -> ToWs_Req_Bus_Sig1/1  "<testSig_Epm_nEng>"
  BS/2 -> ToWs_Req_Bus_Sig2/1  "<testSig_PT_trqLosComp>"
  BS/3 -> ToWs_Req_Bus_Sig3/1  "<testSig_TS_trqDesAcs>"
  BS/4 -> ToWs_Req_Bus_Sig4/1  "<testSig_VehMot_trqDesAcs>"
  BS/5 -> ToWs_Req_Bus_Sig5/1  "<testSig_ESS_trqDesAcs>"
  BS/6 -> ToWs_Req_Bus_Sig6/1  "<testSig_PT_trqResv>"
  BS/7 -> ToWs_Req_Bus_Sig7/1  "<testSig_TS_trqResvAcs>"
  BS/8 -> ToWs_Req_Bus_Sig8/1  "<testSig_VehMot_trqResvAcs>"
  BS/9 -> ToWs_Req_Bus_Sig9/1  "<testSig_ESS_trqResvAcs>"
  BS/10 -> ToWs_Req_Bus_Sig10/1  "<testSig_TS_nMax>"
  BS/11 -> ToWs_Req_Bus_Sig11/1  "<testSig_VehMot_nMaxAcs>"
  BS/12 -> ToWs_Req_Bus_Sig12/1  "<testSig_ESS_nMax>"
  BS/13 -> ToWs_Req_Bus_Sig13/1  "<testSig_TS_nMin>"
  BS/14 -> ToWs_Req_Bus_Sig14/1  "<testSig_VehMot_nMinAcs>"
  BS/15 -> ToWs_Req_Bus_Sig15/1  "<testSig_ESS_nMin>"
  BS/16 -> ToWs_Req_Bus_Sig16/1  "<testSig_TS_nMinAC>"
  BS/17 -> ToWs_Req_Bus_Sig17/1  "<testSig_CoME_trqDesComp>"
  BS/18 -> ToWs_Req_Bus_Sig18/1  "<testSig_CoVeh_trqAcs>"
  BS/19 -> ToWs_Req_Bus_Sig19/1  "<testSig_CoME_trqResv>"
  BS/20 -> ToWs_Req_Bus_Sig20/1  "<testSig_CoME_nMax>"
  BS/21 -> ToWs_Req_Bus_Sig21/1  "<testSig_CoME_nMin>"
  BS/22 -> ToWs_Req_Bus_Sig22/1  "<testSig_CoME_stNSetP>"
  sig_Result_Bus/1 -> BS_Result/1, specifyOutputs/2(sig_Result_Bus)
  BS_Result/1 -> ToWs_Result_Bus_Sig1/1  "<CoME_trqDesComp>"
  BS_Result/2 -> ToWs_Result_Bus_Sig2/1  "<CoVeh_trqAcs>"
  BS_Result/3 -> ToWs_Result_Bus_Sig3/1  "<CoME_trqResv>"
  BS_Result/4 -> ToWs_Result_Bus_Sig4/1  "<CoME_nMax>"
  BS_Result/5 -> ToWs_Result_Bus_Sig5/1  "<CoME_nMin>"
  BS_Result/6 -> ToWs_Result_Bus_Sig6/1  "<CoME_stNSetP>"
  specifyOutputs/1(result) -> result/1

== system TST_CoME_DemCoord/simulationInput/testSignals_R001 ==
  BC : BusCreator  Inputs=22
  spec_CoME_nMax : FromWorkspace  VariableName=testSig_CoME_nMax  Interpolate=off  OutputAfterFinalValue=Holding final value
  spec_CoME_nMin : FromWorkspace  VariableName=testSig_CoME_nMin  Interpolate=off  OutputAfterFinalValue=Holding final value
  spec_CoME_stNSetP : FromWorkspace  VariableName=testSig_CoME_stNSetP  Interpolate=off  OutputAfterFinalValue=Holding final value
  spec_CoME_trqDesComp : FromWorkspace  VariableName=testSig_CoME_trqDesComp  Interpolate=off  OutputAfterFinalValue=Holding final value
  spec_CoME_trqResv : FromWorkspace  VariableName=testSig_CoME_trqResv  Interpolate=off  OutputAfterFinalValue=Holding final value
  spec_CoVeh_trqAcs : FromWorkspace  VariableName=testSig_CoVeh_trqAcs  Interpolate=off  OutputAfterFinalValue=Holding final value
  spec_ESS_nMax : FromWorkspace  VariableName=testSig_ESS_nMax  Interpolate=off  OutputAfterFinalValue=Holding final value
  spec_ESS_nMin : FromWorkspace  VariableName=testSig_ESS_nMin  Interpolate=off  OutputAfterFinalValue=Holding final value
  spec_ESS_trqDesAcs : FromWorkspace  VariableName=testSig_ESS_trqDesAcs  Interpolate=off  OutputAfterFinalValue=Holding final value
  spec_ESS_trqResvAcs : FromWorkspace  VariableName=testSig_ESS_trqResvAcs  Interpolate=off  OutputAfterFinalValue=Holding final value
  spec_Epm_nEng : FromWorkspace  VariableName=testSig_Epm_nEng  Interpolate=off  OutputAfterFinalValue=Holding final value
  spec_PT_trqLosComp : FromWorkspace  VariableName=testSig_PT_trqLosComp  Interpolate=off  OutputAfterFinalValue=Holding final value
  spec_PT_trqResv : FromWorkspace  VariableName=testSig_PT_trqResv  Interpolate=off  OutputAfterFinalValue=Holding final value
  spec_TS_nMax : FromWorkspace  VariableName=testSig_TS_nMax  Interpolate=off  OutputAfterFinalValue=Holding final value
  spec_TS_nMin : FromWorkspace  VariableName=testSig_TS_nMin  Interpolate=off  OutputAfterFinalValue=Holding final value
  spec_TS_nMinAC : FromWorkspace  VariableName=testSig_TS_nMinAC  Interpolate=off  OutputAfterFinalValue=Holding final value
  spec_TS_trqDesAcs : FromWorkspace  VariableName=testSig_TS_trqDesAcs  Interpolate=off  OutputAfterFinalValue=Holding final value
  spec_TS_trqResvAcs : FromWorkspace  VariableName=testSig_TS_trqResvAcs  Interpolate=off  OutputAfterFinalValue=Holding final value
  spec_VehMot_nMaxAcs : FromWorkspace  VariableName=testSig_VehMot_nMaxAcs  Interpolate=off  OutputAfterFinalValue=Holding final value
  spec_VehMot_nMinAcs : FromWorkspace  VariableName=testSig_VehMot_nMinAcs  Interpolate=off  OutputAfterFinalValue=Holding final value
  spec_VehMot_trqDesAcs : FromWorkspace  VariableName=testSig_VehMot_trqDesAcs  Interpolate=off  OutputAfterFinalValue=Holding final value
  spec_VehMot_trqResvAcs : FromWorkspace  VariableName=testSig_VehMot_trqResvAcs  Interpolate=off  OutputAfterFinalValue=Holding final value
  testSignals : Outport
  wires:
  BC/1 -> testSignals/1
  spec_Epm_nEng/1 -> BC/1  "testSig_Epm_nEng"
  spec_PT_trqLosComp/1 -> BC/2  "testSig_PT_trqLosComp"
  spec_TS_trqDesAcs/1 -> BC/3  "testSig_TS_trqDesAcs"
  spec_VehMot_trqDesAcs/1 -> BC/4  "testSig_VehMot_trqDesAcs"
  spec_ESS_trqDesAcs/1 -> BC/5  "testSig_ESS_trqDesAcs"
  spec_PT_trqResv/1 -> BC/6  "testSig_PT_trqResv"
  spec_TS_trqResvAcs/1 -> BC/7  "testSig_TS_trqResvAcs"
  spec_VehMot_trqResvAcs/1 -> BC/8  "testSig_VehMot_trqResvAcs"
  spec_ESS_trqResvAcs/1 -> BC/9  "testSig_ESS_trqResvAcs"
  spec_TS_nMax/1 -> BC/10  "testSig_TS_nMax"
  spec_VehMot_nMaxAcs/1 -> BC/11  "testSig_VehMot_nMaxAcs"
  spec_ESS_nMax/1 -> BC/12  "testSig_ESS_nMax"
  spec_TS_nMin/1 -> BC/13  "testSig_TS_nMin"
  spec_VehMot_nMinAcs/1 -> BC/14  "testSig_VehMot_nMinAcs"
  spec_ESS_nMin/1 -> BC/15  "testSig_ESS_nMin"
  spec_TS_nMinAC/1 -> BC/16  "testSig_TS_nMinAC"
  spec_CoME_trqDesComp/1 -> BC/17  "testSig_CoME_trqDesComp"
  spec_CoVeh_trqAcs/1 -> BC/18  "testSig_CoVeh_trqAcs"
  spec_CoME_trqResv/1 -> BC/19  "testSig_CoME_trqResv"
  spec_CoME_nMax/1 -> BC/20  "testSig_CoME_nMax"
  spec_CoME_nMin/1 -> BC/21  "testSig_CoME_nMin"
  spec_CoME_stNSetP/1 -> BC/22  "testSig_CoME_stNSetP"

== system TST_CoME_DemCoord/simulationInput/testSignals_R002 ==
  BC : BusCreator  Inputs=22
  spec_CoME_nMax : FromWorkspace  VariableName=testSig_CoME_nMax  Interpolate=off  OutputAfterFinalValue=Holding final value
  spec_CoME_nMin : FromWorkspace  VariableName=testSig_CoME_nMin  Interpolate=off  OutputAfterFinalValue=Holding final value
  spec_CoME_stNSetP : FromWorkspace  VariableName=testSig_CoME_stNSetP  Interpolate=off  OutputAfterFinalValue=Holding final value
  spec_CoME_trqDesComp : FromWorkspace  VariableName=testSig_CoME_trqDesComp  Interpolate=off  OutputAfterFinalValue=Holding final value
  spec_CoME_trqResv : FromWorkspace  VariableName=testSig_CoME_trqResv  Interpolate=off  OutputAfterFinalValue=Holding final value
  spec_CoVeh_trqAcs : FromWorkspace  VariableName=testSig_CoVeh_trqAcs  Interpolate=off  OutputAfterFinalValue=Holding final value
  spec_ESS_nMax : FromWorkspace  VariableName=testSig_ESS_nMax  Interpolate=off  OutputAfterFinalValue=Holding final value
  spec_ESS_nMin : FromWorkspace  VariableName=testSig_ESS_nMin  Interpolate=off  OutputAfterFinalValue=Holding final value
  spec_ESS_trqDesAcs : FromWorkspace  VariableName=testSig_ESS_trqDesAcs  Interpolate=off  OutputAfterFinalValue=Holding final value
  spec_ESS_trqResvAcs : FromWorkspace  VariableName=testSig_ESS_trqResvAcs  Interpolate=off  OutputAfterFinalValue=Holding final value
  spec_Epm_nEng : FromWorkspace  VariableName=testSig_Epm_nEng  Interpolate=off  OutputAfterFinalValue=Holding final value
  spec_PT_trqLosComp : FromWorkspace  VariableName=testSig_PT_trqLosComp  Interpolate=off  OutputAfterFinalValue=Holding final value
  spec_PT_trqResv : FromWorkspace  VariableName=testSig_PT_trqResv  Interpolate=off  OutputAfterFinalValue=Holding final value
  spec_TS_nMax : FromWorkspace  VariableName=testSig_TS_nMax  Interpolate=off  OutputAfterFinalValue=Holding final value
  spec_TS_nMin : FromWorkspace  VariableName=testSig_TS_nMin  Interpolate=off  OutputAfterFinalValue=Holding final value
  spec_TS_nMinAC : FromWorkspace  VariableName=testSig_TS_nMinAC  Interpolate=off  OutputAfterFinalValue=Holding final value
  spec_TS_trqDesAcs : FromWorkspace  VariableName=testSig_TS_trqDesAcs  Interpolate=off  OutputAfterFinalValue=Holding final value
  spec_TS_trqResvAcs : FromWorkspace  VariableName=testSig_TS_trqResvAcs  Interpolate=off  OutputAfterFinalValue=Holding final value
  spec_VehMot_nMaxAcs : FromWorkspace  VariableName=testSig_VehMot_nMaxAcs  Interpolate=off  OutputAfterFinalValue=Holding final value
  spec_VehMot_nMinAcs : FromWorkspace  VariableName=testSig_VehMot_nMinAcs  Interpolate=off  OutputAfterFinalValue=Holding final value
  spec_VehMot_trqDesAcs : FromWorkspace  VariableName=testSig_VehMot_trqDesAcs  Interpolate=off  OutputAfterFinalValue=Holding final value
  spec_VehMot_trqResvAcs : FromWorkspace  VariableName=testSig_VehMot_trqResvAcs  Interpolate=off  OutputAfterFinalValue=Holding final value
  testSignals : Outport
  wires:
  BC/1 -> testSignals/1
  spec_Epm_nEng/1 -> BC/1  "testSig_Epm_nEng"
  spec_PT_trqLosComp/1 -> BC/2  "testSig_PT_trqLosComp"
  spec_TS_trqDesAcs/1 -> BC/3  "testSig_TS_trqDesAcs"
  spec_VehMot_trqDesAcs/1 -> BC/4  "testSig_VehMot_trqDesAcs"
  spec_ESS_trqDesAcs/1 -> BC/5  "testSig_ESS_trqDesAcs"
  spec_PT_trqResv/1 -> BC/6  "testSig_PT_trqResv"
  spec_TS_trqResvAcs/1 -> BC/7  "testSig_TS_trqResvAcs"
  spec_VehMot_trqResvAcs/1 -> BC/8  "testSig_VehMot_trqResvAcs"
  spec_ESS_trqResvAcs/1 -> BC/9  "testSig_ESS_trqResvAcs"
  spec_TS_nMax/1 -> BC/10  "testSig_TS_nMax"
  spec_VehMot_nMaxAcs/1 -> BC/11  "testSig_VehMot_nMaxAcs"
  spec_ESS_nMax/1 -> BC/12  "testSig_ESS_nMax"
  spec_TS_nMin/1 -> BC/13  "testSig_TS_nMin"
  spec_VehMot_nMinAcs/1 -> BC/14  "testSig_VehMot_nMinAcs"
  spec_ESS_nMin/1 -> BC/15  "testSig_ESS_nMin"
  spec_TS_nMinAC/1 -> BC/16  "testSig_TS_nMinAC"
  spec_CoME_trqDesComp/1 -> BC/17  "testSig_CoME_trqDesComp"
  spec_CoVeh_trqAcs/1 -> BC/18  "testSig_CoVeh_trqAcs"
  spec_CoME_trqResv/1 -> BC/19  "testSig_CoME_trqResv"
  spec_CoME_nMax/1 -> BC/20  "testSig_CoME_nMax"
  spec_CoME_nMin/1 -> BC/21  "testSig_CoME_nMin"
  spec_CoME_stNSetP/1 -> BC/22  "testSig_CoME_stNSetP"

== system TST_CoME_DemCoord/simulationInput/testSignals_R003 ==
  BC : BusCreator  Inputs=22
  spec_CoME_nMax : FromWorkspace  VariableName=testSig_CoME_nMax  Interpolate=off  OutputAfterFinalValue=Holding final value
  spec_CoME_nMin : FromWorkspace  VariableName=testSig_CoME_nMin  Interpolate=off  OutputAfterFinalValue=Holding final value
  spec_CoME_stNSetP : FromWorkspace  VariableName=testSig_CoME_stNSetP  Interpolate=off  OutputAfterFinalValue=Holding final value
  spec_CoME_trqDesComp : FromWorkspace  VariableName=testSig_CoME_trqDesComp  Interpolate=off  OutputAfterFinalValue=Holding final value
  spec_CoME_trqResv : FromWorkspace  VariableName=testSig_CoME_trqResv  Interpolate=off  OutputAfterFinalValue=Holding final value
  spec_CoVeh_trqAcs : FromWorkspace  VariableName=testSig_CoVeh_trqAcs  Interpolate=off  OutputAfterFinalValue=Holding final value
  spec_ESS_nMax : FromWorkspace  VariableName=testSig_ESS_nMax  Interpolate=off  OutputAfterFinalValue=Holding final value
  spec_ESS_nMin : FromWorkspace  VariableName=testSig_ESS_nMin  Interpolate=off  OutputAfterFinalValue=Holding final value
  spec_ESS_trqDesAcs : FromWorkspace  VariableName=testSig_ESS_trqDesAcs  Interpolate=off  OutputAfterFinalValue=Holding final value
  spec_ESS_trqResvAcs : FromWorkspace  VariableName=testSig_ESS_trqResvAcs  Interpolate=off  OutputAfterFinalValue=Holding final value
  spec_Epm_nEng : FromWorkspace  VariableName=testSig_Epm_nEng  Interpolate=off  OutputAfterFinalValue=Holding final value
  spec_PT_trqLosComp : FromWorkspace  VariableName=testSig_PT_trqLosComp  Interpolate=off  OutputAfterFinalValue=Holding final value
  spec_PT_trqResv : FromWorkspace  VariableName=testSig_PT_trqResv  Interpolate=off  OutputAfterFinalValue=Holding final value
  spec_TS_nMax : FromWorkspace  VariableName=testSig_TS_nMax  Interpolate=off  OutputAfterFinalValue=Holding final value
  spec_TS_nMin : FromWorkspace  VariableName=testSig_TS_nMin  Interpolate=off  OutputAfterFinalValue=Holding final value
  spec_TS_nMinAC : FromWorkspace  VariableName=testSig_TS_nMinAC  Interpolate=off  OutputAfterFinalValue=Holding final value
  spec_TS_trqDesAcs : FromWorkspace  VariableName=testSig_TS_trqDesAcs  Interpolate=off  OutputAfterFinalValue=Holding final value
  spec_TS_trqResvAcs : FromWorkspace  VariableName=testSig_TS_trqResvAcs  Interpolate=off  OutputAfterFinalValue=Holding final value
  spec_VehMot_nMaxAcs : FromWorkspace  VariableName=testSig_VehMot_nMaxAcs  Interpolate=off  OutputAfterFinalValue=Holding final value
  spec_VehMot_nMinAcs : FromWorkspace  VariableName=testSig_VehMot_nMinAcs  Interpolate=off  OutputAfterFinalValue=Holding final value
  spec_VehMot_trqDesAcs : FromWorkspace  VariableName=testSig_VehMot_trqDesAcs  Interpolate=off  OutputAfterFinalValue=Holding final value
  spec_VehMot_trqResvAcs : FromWorkspace  VariableName=testSig_VehMot_trqResvAcs  Interpolate=off  OutputAfterFinalValue=Holding final value
  testSignals : Outport
  wires:
  BC/1 -> testSignals/1
  spec_Epm_nEng/1 -> BC/1  "testSig_Epm_nEng"
  spec_PT_trqLosComp/1 -> BC/2  "testSig_PT_trqLosComp"
  spec_TS_trqDesAcs/1 -> BC/3  "testSig_TS_trqDesAcs"
  spec_VehMot_trqDesAcs/1 -> BC/4  "testSig_VehMot_trqDesAcs"
  spec_ESS_trqDesAcs/1 -> BC/5  "testSig_ESS_trqDesAcs"
  spec_PT_trqResv/1 -> BC/6  "testSig_PT_trqResv"
  spec_TS_trqResvAcs/1 -> BC/7  "testSig_TS_trqResvAcs"
  spec_VehMot_trqResvAcs/1 -> BC/8  "testSig_VehMot_trqResvAcs"
  spec_ESS_trqResvAcs/1 -> BC/9  "testSig_ESS_trqResvAcs"
  spec_TS_nMax/1 -> BC/10  "testSig_TS_nMax"
  spec_VehMot_nMaxAcs/1 -> BC/11  "testSig_VehMot_nMaxAcs"
  spec_ESS_nMax/1 -> BC/12  "testSig_ESS_nMax"
  spec_TS_nMin/1 -> BC/13  "testSig_TS_nMin"
  spec_VehMot_nMinAcs/1 -> BC/14  "testSig_VehMot_nMinAcs"
  spec_ESS_nMin/1 -> BC/15  "testSig_ESS_nMin"
  spec_TS_nMinAC/1 -> BC/16  "testSig_TS_nMinAC"
  spec_CoME_trqDesComp/1 -> BC/17  "testSig_CoME_trqDesComp"
  spec_CoVeh_trqAcs/1 -> BC/18  "testSig_CoVeh_trqAcs"
  spec_CoME_trqResv/1 -> BC/19  "testSig_CoME_trqResv"
  spec_CoME_nMax/1 -> BC/20  "testSig_CoME_nMax"
  spec_CoME_nMin/1 -> BC/21  "testSig_CoME_nMin"
  spec_CoME_stNSetP/1 -> BC/22  "testSig_CoME_stNSetP"

== system TST_CoME_DemCoord/simulationInput/testSignals_R004 ==
  BC : BusCreator  Inputs=22
  spec_CoME_nMax : FromWorkspace  VariableName=testSig_CoME_nMax  Interpolate=off  OutputAfterFinalValue=Holding final value
  spec_CoME_nMin : FromWorkspace  VariableName=testSig_CoME_nMin  Interpolate=off  OutputAfterFinalValue=Holding final value
  spec_CoME_stNSetP : FromWorkspace  VariableName=testSig_CoME_stNSetP  Interpolate=off  OutputAfterFinalValue=Holding final value
  spec_CoME_trqDesComp : FromWorkspace  VariableName=testSig_CoME_trqDesComp  Interpolate=off  OutputAfterFinalValue=Holding final value
  spec_CoME_trqResv : FromWorkspace  VariableName=testSig_CoME_trqResv  Interpolate=off  OutputAfterFinalValue=Holding final value
  spec_CoVeh_trqAcs : FromWorkspace  VariableName=testSig_CoVeh_trqAcs  Interpolate=off  OutputAfterFinalValue=Holding final value
  spec_ESS_nMax : FromWorkspace  VariableName=testSig_ESS_nMax  Interpolate=off  OutputAfterFinalValue=Holding final value
  spec_ESS_nMin : FromWorkspace  VariableName=testSig_ESS_nMin  Interpolate=off  OutputAfterFinalValue=Holding final value
  spec_ESS_trqDesAcs : FromWorkspace  VariableName=testSig_ESS_trqDesAcs  Interpolate=off  OutputAfterFinalValue=Holding final value
  spec_ESS_trqResvAcs : FromWorkspace  VariableName=testSig_ESS_trqResvAcs  Interpolate=off  OutputAfterFinalValue=Holding final value
  spec_Epm_nEng : FromWorkspace  VariableName=testSig_Epm_nEng  Interpolate=off  OutputAfterFinalValue=Holding final value
  spec_PT_trqLosComp : FromWorkspace  VariableName=testSig_PT_trqLosComp  Interpolate=off  OutputAfterFinalValue=Holding final value
  spec_PT_trqResv : FromWorkspace  VariableName=testSig_PT_trqResv  Interpolate=off  OutputAfterFinalValue=Holding final value
  spec_TS_nMax : FromWorkspace  VariableName=testSig_TS_nMax  Interpolate=off  OutputAfterFinalValue=Holding final value
  spec_TS_nMin : FromWorkspace  VariableName=testSig_TS_nMin  Interpolate=off  OutputAfterFinalValue=Holding final value
  spec_TS_nMinAC : FromWorkspace  VariableName=testSig_TS_nMinAC  Interpolate=off  OutputAfterFinalValue=Holding final value
  spec_TS_trqDesAcs : FromWorkspace  VariableName=testSig_TS_trqDesAcs  Interpolate=off  OutputAfterFinalValue=Holding final value
  spec_TS_trqResvAcs : FromWorkspace  VariableName=testSig_TS_trqResvAcs  Interpolate=off  OutputAfterFinalValue=Holding final value
  spec_VehMot_nMaxAcs : FromWorkspace  VariableName=testSig_VehMot_nMaxAcs  Interpolate=off  OutputAfterFinalValue=Holding final value
  spec_VehMot_nMinAcs : FromWorkspace  VariableName=testSig_VehMot_nMinAcs  Interpolate=off  OutputAfterFinalValue=Holding final value
  spec_VehMot_trqDesAcs : FromWorkspace  VariableName=testSig_VehMot_trqDesAcs  Interpolate=off  OutputAfterFinalValue=Holding final value
  spec_VehMot_trqResvAcs : FromWorkspace  VariableName=testSig_VehMot_trqResvAcs  Interpolate=off  OutputAfterFinalValue=Holding final value
  testSignals : Outport
  wires:
  BC/1 -> testSignals/1
  spec_Epm_nEng/1 -> BC/1  "testSig_Epm_nEng"
  spec_PT_trqLosComp/1 -> BC/2  "testSig_PT_trqLosComp"
  spec_TS_trqDesAcs/1 -> BC/3  "testSig_TS_trqDesAcs"
  spec_VehMot_trqDesAcs/1 -> BC/4  "testSig_VehMot_trqDesAcs"
  spec_ESS_trqDesAcs/1 -> BC/5  "testSig_ESS_trqDesAcs"
  spec_PT_trqResv/1 -> BC/6  "testSig_PT_trqResv"
  spec_TS_trqResvAcs/1 -> BC/7  "testSig_TS_trqResvAcs"
  spec_VehMot_trqResvAcs/1 -> BC/8  "testSig_VehMot_trqResvAcs"
  spec_ESS_trqResvAcs/1 -> BC/9  "testSig_ESS_trqResvAcs"
  spec_TS_nMax/1 -> BC/10  "testSig_TS_nMax"
  spec_VehMot_nMaxAcs/1 -> BC/11  "testSig_VehMot_nMaxAcs"
  spec_ESS_nMax/1 -> BC/12  "testSig_ESS_nMax"
  spec_TS_nMin/1 -> BC/13  "testSig_TS_nMin"
  spec_VehMot_nMinAcs/1 -> BC/14  "testSig_VehMot_nMinAcs"
  spec_ESS_nMin/1 -> BC/15  "testSig_ESS_nMin"
  spec_TS_nMinAC/1 -> BC/16  "testSig_TS_nMinAC"
  spec_CoME_trqDesComp/1 -> BC/17  "testSig_CoME_trqDesComp"
  spec_CoVeh_trqAcs/1 -> BC/18  "testSig_CoVeh_trqAcs"
  spec_CoME_trqResv/1 -> BC/19  "testSig_CoME_trqResv"
  spec_CoME_nMax/1 -> BC/20  "testSig_CoME_nMax"
  spec_CoME_nMin/1 -> BC/21  "testSig_CoME_nMin"
  spec_CoME_stNSetP/1 -> BC/22  "testSig_CoME_stNSetP"
